simulink model "complete_state_observer"  (R2020b)
settings: Solver=VariableStepAuto  StartTime=0.0  StopTime=10.0  RelTol=1e-3
settings Model: Creator=petir  LastModifiedBy=petir

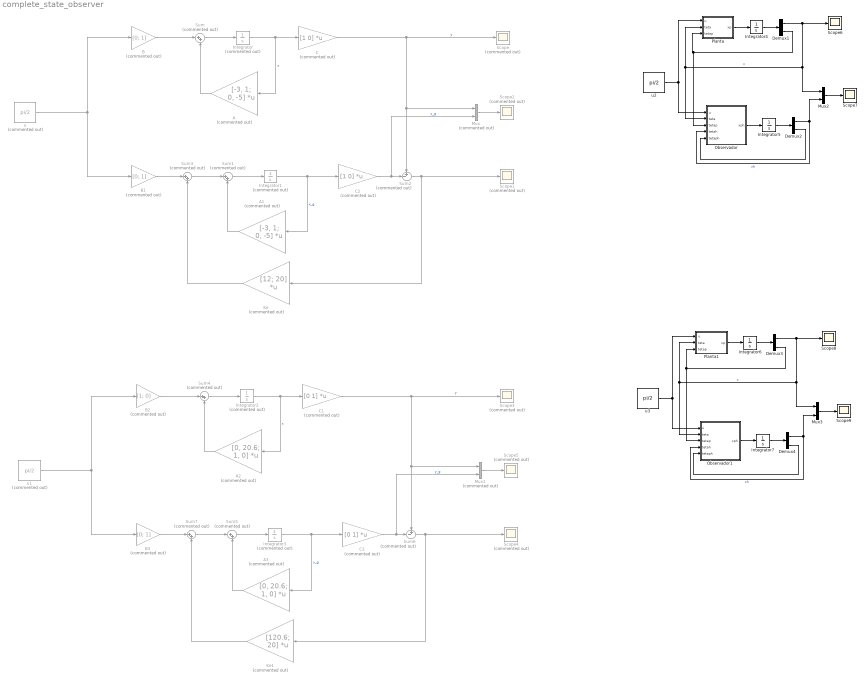
== system complete_state_observer ==
  A : Gain  Commented=on  Gain=[-3, 1; 0, -5]  Multiplication=Matrix(K*u)
  A1 : Gain  Commented=on  Gain=[-3, 1; 0, -5]  Multiplication=Matrix(K*u)
  A2 : Gain  Commented=on  Gain=[0, 20.6; 1, 0]  Multiplication=Matrix(K*u)
  A3 : Gain  Commented=on  Gain=[0, 20.6; 1, 0]  Multiplication=Matrix(K*u)
  B : Gain  Commented=on  Gain=[0; 1]
  B1 : Gain  Commented=on  Gain=[0; 1]
  B2 : Gain  Commented=on  Gain=[1; 0]
  B3 : Gain  Commented=on  Gain=[0; 1]
  C : Gain  Commented=on  Gain=[1 0]  Multiplication=Matrix(K*u) (u vector)
  C1 : Gain  Commented=on  Gain=[0 1]  Multiplication=Matrix(K*u) (u vector)
  C2 : Gain  Commented=on  Gain=[1 0]  Multiplication=Matrix(K*u) (u vector)
  C3 : Gain  Commented=on  Gain=[0 1]  Multiplication=Matrix(K*u) (u vector)
  Demux{1..4} (4 alike) : Demux  Outputs=2
  Integrator{,1..3} (4 alike) : Integrator  Commented=on
  Integrator{4..7} (4 alike) : Integrator
  Ke : Gain  Commented=on  Gain=[12; 20]  Multiplication=Matrix(K*u)
  Ke1 : Gain  Commented=on  Gain=[120.6; 20]  Multiplication=Matrix(K*u)
  Mux : Mux  Commented=on  Inputs=2
  Mux1 : Mux  Commented=on  Inputs=2
  Mux2 : Mux  Inputs=2
  Mux3 : Mux  Inputs=2
  Observador : MATLAB Function  TreatAsAtomicUnit=on
  Observador1 : MATLAB Function  TreatAsAtomicUnit=on
  Planta : MATLAB Function  TreatAsAtomicUnit=on
  Planta1 : MATLAB Function  TreatAsAtomicUnit=on
  Scope{,1..5} (6 alike) : Scope  Commented=on
  Scope{6..9} (4 alike) : Scope
  Sum{,1,3..5,7} (6 alike) : Sum  Commented=on  Inputs=|++
  Sum2 : Sum  Commented=on  Inputs=+-|
  Sum6 : Sum  Commented=on  Inputs=+-|
  u : Constant  Commented=on  Value=pi/2  VectorParams1D=off
  u1 : Constant  Commented=on  Value=pi/2  VectorParams1D=off
  u2 : Constant  Value=pi/2  VectorParams1D=off
  u3 : Constant  Value=pi/2  VectorParams1D=off
  wires:
  u/1 -> B1/1, B/1
  B/1 -> Sum/1
  Sum/1 -> Integrator/1
  A/1 -> Sum/2
  Integrator/1 -> C/1, A/1  "x"
  C/1 -> Mux/1, Sum2/1, Scope/1  "y"
  Integrator1/1 -> C2/1, A1/1  "x_g"
  A1/1 -> Sum1/2
  Sum1/1 -> Integrator1/1
  C2/1 -> Mux/2, Sum2/2  "y_g"
  Sum2/1 -> Scope1/1, Ke/1
  Ke/1 -> Sum3/2
  Sum3/1 -> Sum1/1
  B1/1 -> Sum3/1
  Mux/1 -> Scope2/1
  Sum5/1 -> Integrator3/1
  A3/1 -> Sum5/2
  Sum6/1 -> Scope4/1, Ke1/1
  Sum7/1 -> Sum5/1
  Ke1/1 -> Sum7/2
  Integrator3/1 -> C3/1, A3/1  "x_g"
  C1/1 -> Mux1/1, Sum6/1, Scope3/1  "y"
  C3/1 -> Mux1/2, Sum6/2  "y_g"
  Integrator2/1 -> C1/1, A2/1  "x"
  A2/1 -> Sum4/2
  Sum4/1 -> Integrator2/1
  B3/1 -> Sum7/1
  B2/1 -> Sum4/1
  u1/1 -> B3/1, B2/1
  Mux1/1 -> Scope5/1
  Integrator4/1 -> Demux1/1
  Planta/1(xp) -> Integrator4/1
  Demux1/2 -> Observador/3(tetap), Planta/3(tetap)
  Demux1/1 -> Scope6/1, Mux2/1, Observador/2(teta), Planta/2(teta)  "x"
  u2/1 -> Observador/1(u), Planta/1(u)
  Observador/1(xph) -> Integrator5/1
  Integrator5/1 -> Demux2/1
  Demux2/2 -> Observador/5(tetaph)
  Demux2/1 -> Mux2/2, Observador/4(tetah)  "xh"
  Mux2/1 -> Scope7/1
  Observador1/1(xph) -> Integrator7/1
  Demux3/2 -> Observador1/3(tetap), Planta1/3(tetap)
  Integrator6/1 -> Demux3/1
  Demux3/1 -> Scope8/1, Mux3/1, Observador1/2(teta), Planta1/2(teta)  "x"
  Demux4/2 -> Observador1/5(tetaph)
  Demux4/1 -> Mux3/2, Observador1/4(tetah)  "xh"
  Planta1/1(xp) -> Integrator6/1
  Integrator7/1 -> Demux4/1
  Mux3/1 -> Scope9/1
  u3/1 -> Observador1/1(u), Planta1/1(u)

== matlab function complete_state_observer/Observador ==
  data: u input; xph output; teta input; tetap input; tetah input; tetaph input
function xph = fcn(u, teta, tetap, tetah, tetaph)
A = [-3, 1; 0, -5];
B = [0; 1];
C = [1, 0];
K = [12; 20];

% Observador
xh = [tetah; tetaph];
x = [teta; tetap];

y = C * x;
yh = C *xh;
xph = A * xh + B * u + K *(y - yh);

== matlab function complete_state_observer/Planta ==
  data: u input; xp output; teta input; tetap input
function xp = fcn(u, teta, tetap)

A = [-3, 1; 0, -5];
B = [0; 1];

% Planta
x = [teta; tetap];
xp = A*x + B*u;

== matlab function complete_state_observer/Observador1 ==
  data: u input; xph output; teta input; tetap input; tetah input; tetaph input
function xph = fcn(u, teta, tetap, tetah, tetaph)
A = [0, 20.6; 1, 0];
B = [0; 1];
C = [0 1];
K = [120.6; 20];

% Observador
xh = [tetah; tetaph];
x = [teta; tetap];

y = C * x;
yh = C *xh;
xph = A * xh + B * u + K * (y - yh);

== matlab function complete_state_observer/Planta1 ==
  data: u input; xp output; teta input; tetap input
function xp = fcn(u, teta, tetap)

A = [0, 20.6; 1, 0];
B = [0; 1];

% Planta
x = [teta; tetap];
xp = A*x + B*u;
